simulink model "test_com_SensorFusion_SF_D4_ukf"  (R2019b)
settings: Solver=FixedStepDiscrete  StartTime=0  StopTime=stop  FixedStep=0.001  RelTol=1e-3
undefined symbols (not defined in the file or in its folder): breakpoints_camber_posZ, breakpoints_camber_RollAngle, BxTM, ByTM, camber_posZ_rear, camber_RollAngle_front, camber_RollAngle_rear, CxTM, CyTM, enable_kalman_standing, enable_simpleTireLoad_pGL, enable_v2o_direct, g, gamma_stat_front, gamma_stat_rear, gearbox_ratio, l_F, l_R, m_sprung, m_unsprung_quarter, mag_calib_front_center, mag_calib_front_compmatrix, mag_calib_rear_center, mag_calib_rear_compmatrix, should_be_in_theSensorFusion, switch_lat_accel_tireloadestimE8, switch_rocker_direction_FL, switch_rocker_direction_FR, switch_rocker_direction_RL, switch_rocker_direction_RR, switch_VelYcalculation_pSF, testStart_VelX_pSF, testVelY_pSF, tire_r_dyn, track_angle_front, track_width_front, track_width_rear, v2o_x, wheel_kinematics_breakpoints, wheel_kinematics_FL_data, wheel_kinematics_FR_data, wheelbase, x9DFrontX, x9DFrontY, x9DRearX, x9DRearY
libraries: SignalProcessingSensorFusionLib x30, simulink x9
(part 7 of 9)

== matlab function test_com_SensorFusion_SF_D4_ukf/Subsystem14/SensorFusion_E10/Sturzberechnung2/MATLAB Function ==
  data: PosZ input; Camber_PosZ_front output; Camber_PosZ_rear output
function [Camber_PosZ_front, Camber_PosZ_rear] = fcn(PosZ)
Camber_PosZ_front=max(interp1([-25 -22.50 -20.00 -17.50 -15.00 -12.50 -10.00 -7.50 ...
    -5.00 -2.50 0.00 2.50 5.00 7.50 10.00 12.50 15.00 17.50 20.00 22.50 25.00 ], ...
    [-0.83 -0.74 -0.65 -0.56 -0.47 -0.39 -0.30 -0.23 -0.15 -0.07 0.00 0.07 0.14 0.20 ...
    0.27 0.33 0.39 0.44 0.50 0.55 0.60], PosZ,'spline'));
Camber_PosZ_rear=max(interp1([-25 -22.50 -20.00 -17.50 -15.00 -12.50 -10.00 -7.50 ...
    -5.00 -2.50 0.00 2.50 5.00 7.50 10.00 12.50 15.00 17.50 20.00 22.50 25.00],...
    [-0.64 -0.57 -0.50 -0.44 -0.37 -0.30 -0.24 -0.18 -0.12 -0.06 0.00 0.06 0.11 ...
    0.17 0.22 0.27 0.32 0.37 0.41 0.46 0.50], PosZ,'spline'));

end

== matlab function test_com_SensorFusion_SF_D4_ukf/Subsystem14/SensorFusion_E10/Subsystem/TireLoadEstimationE8/tireload estimator  ==
  settings: updateMethod=DISCRETE  sampleTime=0.002
  data: u_in input single; z input single; x_hat output single; m_sprung parameter single; m_unsprung_quarter parameter single; J_Sxx parameter single; J_Syy parameter single; l_R parameter single; l_F parameter single; wheelbase parameter single; track_width_front parameter single; track_width_rear parameter single; h_aero parameter single; g parameter single; rho_air parameter single; h_cg parameter single; cdA parameter single; y output single; P_diag output single; offset output single; lp output single; clA_front parameter single; clA_rear parameter single; motion_ratio_front parameter single; motion_ratio_rear parameter single; motion_ratio_heave_front parameter single; motion_ratio_heave_rear parameter single; motion_ratio_roll_front parameter single; motion_ratio_roll_rear parameter single; spring_stiff_heave_front parameter single; spring_stiff_heave_rear parameter single; damp_coef_heave_front_push parameter single; damp_coef_heave_front_pull parameter single; damp_coef_heave_rear_push parameter single; damp_coef_heave_rear_pull parameter single; spring_stiff_roll_front parameter single; spring_stiff_roll_rear parameter single; damp_coef_roll_front_push parameter single; damp_coef_roll_front_pull parameter single; damp_coef_roll_rear_push parameter single; damp_coef_roll_rear_pull parameter single
function [x_hat, y, P_diag, offset, lp]  = fcn(u_in, z,...
                           m_sprung, m_unsprung_quarter, J_Sxx, J_Syy,...
                           l_R, l_F, wheelbase, track_width_front, track_width_rear, h_aero,...
                           g, rho_air,...
                           h_cg, cdA, clA_front, clA_rear, ...
                            motion_ratio_front, motion_ratio_rear,...
                            motion_ratio_heave_front, motion_ratio_heave_rear,...
                            motion_ratio_roll_front, motion_ratio_roll_rear,...
                           spring_stiff_heave_front, spring_stiff_heave_rear,...
                           damp_coef_heave_front_push, damp_coef_heave_front_pull,...
                           damp_coef_heave_rear_push, damp_coef_heave_rear_pull,...
                           spring_stiff_roll_front, spring_stiff_roll_rear,...
                           damp_coef_roll_front_push, damp_coef_roll_front_pull,...
                           damp_coef_roll_rear_push, damp_coef_roll_rear_pull)

% x    = [z; z_dot; phi; phi_dot; theta; theta_dot];
% u_in = [a_x; a_y; v];
% u    = [a_x; a_y; g; F_aerox; F_aeroFz; F_aeroRz];
% z    = [z; phiF; phiR; theta];
% y    = [tireloadFL; tireloadFR; tireloadRL; tireloadRR];

persistent P x t

% Initialisierung
if isempty(P)
    %Initial state / Initialwerte Zustandsvektor
    x = single([0; 0; 0; 0; 0; 0; 0; 0; 0; 0]);  
    
    %Initial uncertainty / Initialwerte Koviarianzatrix 
    P = single(diag([0; 0; 0; 0; 0; 0; 0; 0; 0; 0]));
    
    %Initial timer / Initialiserung Zähler
    t = single(0);
end

dt    = 0.001;                                 %Time step / Zeitschritt
I     = eye(10);                               %Identity matrix / Einheitsmatrix

% MonoShock Auswahl Druck/Zug-Stufe
if x(6)*l_F + x(2) < 0  %Vorne Druck
    k_msF =2759;% = damp_coef_heave_front_push;
else                    %Vorne Zug
    k_msF =3941;%= damp_coef_heave_front_pull;
end

if x(6)*l_R + x(2) > 0  %Hinten Druck
    k_msR =4137;%= damp_coef_heave_rear_pull;
else                    %Hinten Zug
    k_msR =2869;%= damp_coef_heave_rear_push;
end


% Rolldämpfer Auswahl Druck/Zug-Stufe
if x(4) < 0             % if Bedingung muss überprüft werden!
    k_rdF =1860;%= damp_coef_roll_front_push;
    k_rdR =1876;%= damp_coef_roll_rear_push;
else
    k_rdF =1860;%= damp_coef_roll_front_pull;
    k_rdR =1876;%= damp_coef_roll_rear_pull; 
end

% Aerokräfte
F_aeroFz     = 0.5 * rho_air * clA_front * u_in(3)^2 ;
F_aeroRz     = 0.5 *  rho_air * clA_rear * u_in(3)^2 ;
F_aerox      = 0.5 *  rho_air * cdA   * u_in(3)^2 ;

% Systemdynamik
a21 = -4 * ( motion_ratio_heave_front^2*spring_stiff_heave_front + motion_ratio_heave_rear^2*spring_stiff_heave_rear ) / m_sprung;
a22 = -4 * ( motion_ratio_heave_front^2*k_msF + motion_ratio_heave_front^2*k_msR ) / m_sprung;
a25 =  4 * ( l_F*motion_ratio_heave_front^2*spring_stiff_heave_front - l_R*motion_ratio_heave_rear^2*spring_stiff_heave_rear ) / m_sprung;
a26 =  4 * ( l_F*motion_ratio_heave_front^2*k_msF - l_R*motion_ratio_heave_rear^2*k_msR ) / m_sprung;
a43 = -( track_width_front^2*motion_ratio_roll_front^2*spring_stiff_roll_front + track_width_rear^2*motion_ratio_roll_rear^2*spring_stiff_roll_rear ) / J_Sxx;
a44 = -( track_width_front^2*motion_ratio_roll_front^2*k_rdF + track_width_rear^2*motion_ratio_roll_rear^2*k_rdR ) / J_Sxx;
a61 =  4 * ( l_F*motion_ratio_heave_front^2*spring_stiff_heave_front - l_R*motion_ratio_heave_rear^2*spring_stiff_heave_rear ) / J_Syy;
a62 =  4 * ( l_F*motion_ratio_heave_front^2*k_msF - l_R*motion_ratio_heave_rear^2*k_msR ) / J_Syy;
a65 = -4 * ( l_F^2*motion_ratio_heave_front^2*spring_stiff_heave_front + l_R^2*motion_ratio_heave_rear^2*spring_stiff_heave_rear ) / J_Syy;
a66 = -4 * ( l_F^2*motion_ratio_heave_front^2*k_msF + l_R^2*motion_ratio_heave_rear^2*k_msR ) / J_Syy;

A = [  0,   1,   0,   0,   0,   0,  0,   0,   0,   0;
     a21, a22,   0,   0, a25, a26,  0,   0,   0,   0;
       0,   0,   0,   1,   0,   0,  0,   0,   0,   0;
       0,   0, a43, a44,   0,   0,  0,   0,   0,   0;
       0,   0,   0,   0,   0,   1,  0,   0,   0,   0;
     a61, a62,   0,   0, a65, a66,  0,   0,   0,   0;
       0,   0,   0,   0,   0,   0,  0,   0,   0,   0;
       0,   0,   0,   0,   0,   0,  0,   0,   0,   0;
       0,   0,   0,   0,   0,   0,  0,   0,   0,   0;
       0,   0,   0,   0,   0,   0,  0,   0,   0,   0];

b25 =  1 / m_sprung;
b26 =  1 / m_sprung;
b42 =  h_cg * m_sprung / J_Sxx;
b61 = -h_cg * m_sprung / J_Syy;
b64 =  h_aero / J_Syy;
b65 = -l_F / J_Syy;
b66 =  l_R / J_Syy;

B = [  0,   0,   0,   0,   0;
       0,   0,   0, b25, b26;
       0,   0,   0,   0,   0;
       0, b42,   0,   0,   0;
       0,   0,   0,   0,   0;
     b61,   0, b64, b65, b66;
       0,   0,   0,   0,   0;
       0,   0,   0,   0,   0;
       0,   0,   0,   0,   0;
       0,   0,   0,   0,   0];                          

% RICHTUNG VON F_aerox CHECKEN!!!
u = [-u_in(1); u_in(2); -F_aerox; -F_aeroFz; -F_aeroRz];


% Measurement function / Messmatrix
H = [-1/motion_ratio_front, 0,  track_width_front/motion_ratio_front, 0,  l_F/motion_ratio_front, 0, 1, 0, 0, 0; 
     -1/motion_ratio_front, 0, -track_width_front/motion_ratio_front, 0,  l_F/motion_ratio_front, 0, 0, 1, 0, 0;
     -1/motion_ratio_rear, 0,  track_width_rear/motion_ratio_rear, 0, -l_R/motion_ratio_rear, 0, 0, 0, 1, 0;
     -1/motion_ratio_rear, 0, -track_width_rear/motion_ratio_rear, 0, -l_R/motion_ratio_rear, 0, 0, 0, 0, 1];

% Measurement noise covariance / Messrauschkovarianzmatrix
R = diag([1; 1; 1; 1]);

% Process Noise Covariance / Prozessrauschkovarianzmatrix 
if abs(u_in(3)) <= 0.5                      %keine statische Offsetzschätzung
        q_offset = 0;
elseif abs(u_in(3)) > 0.1 && t < 3          %schnelle Anfangsschätzung
        q_offset = 1e-8;
        t = t + dt;
else                                        %langsame Detailanpassung
        q_offset = 1e-16;
end
Q = diag([1e-9; 1e-9; 1e-9; 1e-9; 6e-9; 6e-9; q_offset; q_offset; q_offset; q_offset]);

% Prädiktorschritt
x = x + dt * ( A * x + B * u );
P = ( I + dt * A ) * P * ( I + dt * A )' + Q;

% Korrektorschritt
K = P * H' / ( H * P * H' + R );            %Filter-Matrix (Kalman-Gain)
x = x + K * ( z - H * x );                  %aktualisieren des Systemzustands
P = ( I - K * H ) * P;                      %aktualisieren der Kovarianz

% Ausgang
C = [2*motion_ratio_heave_front^2*spring_stiff_heave_front, 2*motion_ratio_heave_front^2*k_msF, -track_width_front*motion_ratio_roll_front^2*spring_stiff_roll_front, -track_width_front*motion_ratio_roll_front^2*k_rdF, -2*l_F*motion_ratio_heave_front^2*spring_stiff_heave_front, -2*l_F*motion_ratio_heave_front^2*k_msF, 0, 0, 0, 0;
     2*motion_ratio_heave_front^2*spring_stiff_heave_front, 2*motion_ratio_heave_front^2*k_msF,  track_width_front*motion_ratio_roll_front^2*spring_stiff_roll_front,  track_width_front*motion_ratio_roll_front^2*k_rdF, -2*l_F*motion_ratio_heave_front^2*spring_stiff_heave_front, -2*l_F*motion_ratio_heave_front^2*k_msF, 0, 0, 0, 0;
     2*motion_ratio_heave_rear^2*spring_stiff_heave_rear, 2*motion_ratio_heave_rear^2*k_msR, -track_width_rear*motion_ratio_roll_rear^2*spring_stiff_roll_rear, -track_width_rear*motion_ratio_roll_rear^2*k_rdR,  2*l_R*motion_ratio_heave_rear^2*spring_stiff_heave_rear,  2*l_R*motion_ratio_heave_rear^2*k_msR, 0, 0, 0, 0;
     2*motion_ratio_heave_rear^2*spring_stiff_heave_rear, 2*motion_ratio_heave_rear^2*k_msR,  track_width_rear*motion_ratio_roll_rear^2*spring_stiff_roll_rear,  track_width_rear*motion_ratio_roll_rear^2*k_rdR,  2*l_R*motion_ratio_heave_rear^2*spring_stiff_heave_rear,  2*l_R*motion_ratio_heave_rear^2*k_msR, 0, 0, 0, 0];

D = [m_unsprung_quarter + 0.5*m_sprung*l_R/wheelbase; 
     m_unsprung_quarter + 0.5*m_sprung*l_R/wheelbase; 
     m_unsprung_quarter + 0.5*m_sprung*l_F/wheelbase; 
     m_unsprung_quarter + 0.5*m_sprung*l_F/wheelbase]*g;

y = C * x + D;

% Begrenzung der Radlast
for n=1:1:4
    if y(n) > 1800
        y(n) = 1800;
    elseif y(n) < 0
        y(n) = 0;
    end
end

% Ausgabe
os_z     = - 0.5*(motion_ratio_front*x(7)+motion_ratio_front*x(8))*l_R/wheelbase - 0.5*(motion_ratio_rear*x(9)+motion_ratio_rear*x(10))*l_F/wheelbase;  
os_phi  = l_R/wheelbase*( x(7)*motion_ratio_front - x(8)*motion_ratio_front ) / track_width_front + l_F/wheelbase*( x(9)*motion_ratio_rear - x(10)*motion_ratio_rear ) / track_width_rear;
os_theta = ( motion_ratio_front*x(7) + motion_ratio_front*x(8) - motion_ratio_rear*x(9) - motion_ratio_rear*x(10) ) / 2 * wheelbase;

x_hat  = [ x(1) + os_z;
           x(2);
          (x(3) + os_phi)   * 180 / pi;
           x(4)             * 180 / pi;
          (x(5) + os_theta) * 180 / pi;
           x(6)             * 180 / pi];

P_diag = [P(1,1), P(2,2), P(3,3), P(4,4), P(5,5), P(6,6), P(7,7), P(8,8), P(9,9), P(10,10)];
offset = [x(7); x(8); x(9); x(10)];
lp = H * x;

end

== matlab function test_com_SensorFusion_SF_D4_ukf/Subsystem14/SensorFusion_E10/Sturzberechnung2/MATLAB Function1 ==
  data: Camber_RollAngle_front output; Camber_RollAngle_rear output; RollAngle input
function [Camber_RollAngle_front, Camber_RollAngle_rear]= fcn (RollAngle)
Camber_RollAngle_front=max(interp1([-1.50 -1.35 -1.20 -1.05 -0.90 -0.75 -0.60 -0.45 -0.30 -0.15 0.00 ...
0.15 0.30 0.45 0.60 0.75 0.90 1.05 1.20 1.35 1.50], ...
    [1.02 0.92 0.82 0.72 0.62 0.52 0.42 0.31 0.21 0.11 0.00 -0.11 -0.21 -0.32 -0.43 -0.53 -0.64 ...
-0.75 -0.86 -0.97 -1.08], RollAngle,'spline'));
Camber_RollAngle_rear=max(interp1([-1.50 -1.35 -1.20 -1.05 -0.90 -0.75 -0.60 -0.45 -0.30 -0.15 0.00 ...
0.15 0.30 0.45 0.60 0.75 0.90 1.05 1.20 1.35 1.50],...
    [1.11 1.00 0.89 0.78 0.67 0.56 0.45 0.34 0.23 0.11 0.00 -0.12 -0.23 -0.35 -0.46 -0.58 ...
-0.70 -0.81 -0.93 -1.05 -1.17], RollAngle,'spline'));
end

== matlab function test_com_SensorFusion_SF_D4_ukf/Subsystem14/SensorFusion_E10/Subsystem/simpleTireLoadEstimation/MATLAB Function ==
  data: a_x input; F_z_vl output; a_y input; F_z_vr output; F_z_hl output; F_z_hr output
function [F_z_vl, F_z_vr, F_z_hl, F_z_hr] = Radlast_Beschleunigung_e9_SAE(a_x, a_y)
m=240;
g=9.81;
l=1.540;
l_v=0.796;
l_h=l-l_v;
h_s=0.2648;
b_v=0.6*2;
b_h=0.6*2;
F_z_vl=single(0);
F_z_vr=single(0);
F_z_hl=single(0);
F_z_hr=single(0);
 %m=Fahrzeugmasse; h_s= Schwerpunktshöhe (von SP zu Anbindung von Rods an Radträger); l_h= Abstand von HA zu
 %SP; l_v=Radstand von VA zum SP l=Radstand; a_x=Beschleunigung in x-Richtung; a_y=Beschleunigung
 %in y-Richtung; b_v=Spurbreite vorne;b_h=Spurbreite hinten; 
 
 %EDITIERT, so dass Vorzeichen vor h_s*a_y/(b_v*g) jeweils getauscht wurde

m_ges_f= m * (l-l_v)/l;
m_ges_r= m * l_v/l;
Delta_TireLoad_x = m * (h_s/(2*l))*a_x; %die 2 hier ist in E7 Radlastschätzer nicht so drin
%{ TireLoad = [...
%    m_ges_f *(0.5*g + (h_s/b_v)* a_y) - Delta_TireLoad_x ...
%    m_ges_f *(0.5*g - (h_s/b_v)* a_y) - Delta_TireLoad_x ...
%    m_ges_r *(0.5*g + (h_s/b_h)* a_y) + Delta_TireLoad_x ...
%    m_ges_r *(0.5*g - (h_s/b_h)* a_y) + Delta_TireLoad_x];
%}

SiL_WheelStates = [ ...
    m*(l_h*g-h_s*a_x)*(0.5+(h_s*a_y/(b_v*g)))/l;
    m*(l_h*g-h_s*a_x)*(0.5-(h_s*a_y/(b_v*g)))/l;
    m*(l_v*g+h_s*a_x)*(0.5+(h_s*a_y/(b_h*g)))/l;
    m*(l_v*g+h_s*a_x)*(0.5-(h_s*a_y/(b_h*g)))/l
    ];
if SiL_WheelStates(1)<0
    F_z_vl = single(0);
else
    F_z_vl = SiL_WheelStates(1);
end

if SiL_WheelStates(2)<0
    F_z_vr = single(0);
else
    F_z_vr = SiL_WheelStates(2);
end

if SiL_WheelStates(3)<0
    F_z_hl = single(0);
else
    F_z_hl = SiL_WheelStates(3);
end

if SiL_WheelStates(4)<0
    F_z_hr = single(0);
else
    F_z_hr = SiL_WheelStates(4);
end

end

== matlab function test_com_SensorFusion_SF_D4_ukf/Subsystem14/SensorFusion_E10/TireModel_simplePacejka1 ==
  data: TireLoad input; TireSlipLong input; TireLoadEff output; TireForceLong output; TireSlipAngle input; mux_nominal input; TireForceLat output; l_F parameter; l_R parameter; wheelbase parameter; m_unsprung_quarter parameter; m_sprung parameter; BxTM parameter; ByTM parameter; CyTM parameter; CxTM parameter; g parameter
function [TireLoadEff, TireForceLong, TireForceLat] = TireModel_simplePacejka(TireLoad, TireSlipLong, TireSlipAngle, ...
    mux_nominal, l_F, l_R, wheelbase, m_unsprung_quarter, m_sprung, BxTM, ByTM, CyTM, CxTM, g)
%% set variables
Fz = TireLoad;
s_long = TireSlipLong;
s_lat = tan(TireSlipAngle); % sin???
dim_wheel = size(TireLoad);

Fx_eff = zeros(dim_wheel);
Fy_eff = zeros(dim_wheel);
Fxy_res  = zeros(dim_wheel);

e = 0.001;

%% set parameters

ez = 0.05; %0.05 richtwert dictonary
mu_x = mux_nominal;   % aus settings herführen
mu_y = 1.6;   % oder eins? 


%% calculate 
s_res = sqrt(s_long.^2 + s_lat.^2); % nominated total tire slips

Fznull_FL= 0.5*g*l_R/wheelbase*m_sprung+g*m_unsprung_quarter;
Fznull_FR= 0.5*g*l_R/wheelbase*m_sprung+g*m_unsprung_quarter;
Fznull_RL= 0.5*g*l_F/wheelbase*m_sprung+g*m_unsprung_quarter;
Fznull_RR= 0.5*g*l_F/wheelbase*m_sprung+g*m_unsprung_quarter;
Fz0=[Fznull_FL; Fznull_FR; Fznull_RL; Fznull_RR];

Fz_eff = Fz.*(1-ez*(Fz./Fz0).^2); % effective tire loads for mu
Dx = Fz_eff*mu_x; % D-terms for long. in Pacejka
Dy = Fz_eff*mu_y; % D-terms for lat. in Pacejka

Fx_stat = Fz_eff*mu_x.* sin( CxTM* atan(BxTM*s_res./mu_x) ); % pure long. tire forces
Fy_stat = Fz_eff*mu_y.* sin( CyTM* atan(ByTM*s_res./mu_y) ); % pure lat. tire forces
% Fx_stat = D_*sin( C_ * atan(B_*s_ - E_*(B_*s_-atan(B_*s_))) ) - sv;
% Fx_stat = D_*sin( C_ * atan(B_*s_ - E_*(B_*s_-atan(B_*s_))) ) - sv;

% combine long. lat. forces
for i = 1:numel(TireLoad)
    if s_res(i) == 0
        Fx_eff(i) = 0;
        Fy_eff(i) = 0;
    else
        Fxy_res(i) = sqrt( (s_long(i)^2*Fx_stat(i)^2+s_lat(i)^2*Fy_stat(i)^2)/(s_res(i)^2) );
        Fx_eff(i) = Fxy_res(i) *(s_long(i)/s_res(i)); % effective long. tire forces
        Fy_eff(i) = Fxy_res(i) *(s_lat(i)/s_res(i)); % effective lat. tire forces
    end
end

% Fxy_res = Fz_eff*mu;

TireLoadEff = single(Fz_eff);
TireForceLong = single(Fx_eff);
TireForceLat = single(Fy_eff);
end

== matlab function test_com_SensorFusion_SF_D4_ukf/Subsystem14/SensorFusion_E10/simpleTireLoadEstimation/MATLAB Function ==
  data: a_x input; F_z_vl output; a_y input; F_z_vr output; F_z_hl output; F_z_hr output
function [F_z_vl, F_z_vr, F_z_hl, F_z_hr] = Radlast_Beschleunigung_e9_SAE(a_x, a_y)
m=240;
g=9.81;
l=1.540;
l_v=0.796;
l_h=l-l_v;
h_s=0.2648;
b_v=0.6*2;
b_h=0.6*2;
F_z_vl=single(0);
F_z_vr=single(0);
F_z_hl=single(0);
F_z_hr=single(0);
 %m=Fahrzeugmasse; h_s= Schwerpunktshöhe (von SP zu Anbindung von Rods an Radträger); l_h= Abstand von HA zu
 %SP; l_v=Radstand von VA zum SP l=Radstand; a_x=Beschleunigung in x-Richtung; a_y=Beschleunigung
 %in y-Richtung; b_v=Spurbreite vorne;b_h=Spurbreite hinten; 
 
 %EDITIERT, so dass Vorzeichen vor h_s*a_y/(b_v*g) jeweils getauscht wurde

m_ges_f= m * (l-l_v)/l;
m_ges_r= m * l_v/l;
Delta_TireLoad_x = m * (h_s/(2*l))*a_x; %die 2 hier ist in E7 Radlastschätzer nicht so drin
%{ TireLoad = [...
%    m_ges_f *(0.5*g + (h_s/b_v)* a_y) - Delta_TireLoad_x ...
%    m_ges_f *(0.5*g - (h_s/b_v)* a_y) - Delta_TireLoad_x ...
%    m_ges_r *(0.5*g + (h_s/b_h)* a_y) + Delta_TireLoad_x ...
%    m_ges_r *(0.5*g - (h_s/b_h)* a_y) + Delta_TireLoad_x];
%}

SiL_WheelStates = [ ...
    m*(l_h*g-h_s*a_x)*(0.5+(h_s*a_y/(b_v*g)))/l;
    m*(l_h*g-h_s*a_x)*(0.5-(h_s*a_y/(b_v*g)))/l;
    m*(l_v*g+h_s*a_x)*(0.5+(h_s*a_y/(b_h*g)))/l;
    m*(l_v*g+h_s*a_x)*(0.5-(h_s*a_y/(b_h*g)))/l
    ];
if SiL_WheelStates(1)<0
    F_z_vl = single(0);
else
    F_z_vl = SiL_WheelStates(1);
end

if SiL_WheelStates(2)<0
    F_z_vr = single(0);
else
    F_z_vr = SiL_WheelStates(2);
end

if SiL_WheelStates(3)<0
    F_z_hl = single(0);
else
    F_z_hl = SiL_WheelStates(3);
end

if SiL_WheelStates(4)<0
    F_z_hr = single(0);
else
    F_z_hr = SiL_WheelStates(4);
end

end

== matlab function test_com_SensorFusion_SF_D4_ukf/Subsystem14/SensorFusion_E10/SensorFusion_E10/Subsystem2/9D_front_measure/MATLAB Function ==
  data: AccX_Sq input; VD_diag_9Dfront output; AccY_Sq input; AccZ_Sq input; RollRate_Sq input; PitchRate_Sq input; YawRate_Sq input

function VD_diag_9Dfront = diag(AccX_Sq, AccY_Sq, AccZ_Sq, RollRate_Sq, PitchRate_Sq, YawRate_Sq)
bad_Sq_counter=single(0);
VD_diag_9Dfront=0;
persistent timestep_counter_old
if isempty(timestep_counter_old)
    timestep_counter_old=0;
end


if AccX_Sq>4
    bad_Sq_counter=bad_Sq_counter+1;
end
if AccY_Sq>4
    bad_Sq_counter=bad_Sq_counter+1;
end
if AccZ_Sq>4
    bad_Sq_counter=bad_Sq_counter+1;
end
if YawRate_Sq>4
    bad_Sq_counter=bad_Sq_counter+1;
end
if RollRate_Sq>4
    bad_Sq_counter=bad_Sq_counter+1;
end
if PitchRate_Sq>4
    bad_Sq_counter=bad_Sq_counter+1;
end

if  bad_Sq_counter>3
    timestep_counter=timestep_counter_old+1;
else 
    timestep_counter=0;
end
if bad_Sq_counter>3 && timestep_counter >4
    VD_diag_9Dfront=1;
end

timestep_counter_old=timestep_counter;

end

== matlab function test_com_SensorFusion_SF_D4_ukf/Subsystem14/SensorFusion_E10/SensorFusion_E10/Subsystem2/9D_rear_measure/MATLAB Function ==
  data: AccX_Sq input; VD_diag_9Drear output; AccY_Sq input; AccZ_Sq input; YawRate_Sq input; PitchRate_Sq input; RollRate_Sq input
function VD_diag_9Drear = diag(AccX_Sq, AccY_Sq, AccZ_Sq, YawRate_Sq, PitchRate_Sq, RollRate_Sq)
bad_Sq_counter=single(0);
VD_diag_9Drear=0;
persistent timestep_counter_old
if isempty(timestep_counter_old)
    timestep_counter_old=0;
end


if AccX_Sq>4
    bad_Sq_counter=bad_Sq_counter+1;
end
if AccY_Sq>4
    bad_Sq_counter=bad_Sq_counter+1;
end
if AccZ_Sq>4
    bad_Sq_counter=bad_Sq_counter+1;
end
if YawRate_Sq>4
    bad_Sq_counter=bad_Sq_counter+1;
end
if RollRate_Sq>4
    bad_Sq_counter=bad_Sq_counter+1;
end
if PitchRate_Sq>4
    bad_Sq_counter=bad_Sq_counter+1;
end

if  bad_Sq_counter>3
    timestep_counter=timestep_counter_old+1;
else 
    timestep_counter=0;
end


if bad_Sq_counter>3 && timestep_counter >4
    VD_diag_9Drear=1;
end

timestep_counter_old=timestep_counter;

end

== matlab function test_com_SensorFusion_SF_D4_ukf/Subsystem14/SensorFusion_E10/SensorFusion_E10/Subsystem2/MATLAB Function1 ==
  data: VD_diag_9Dfront input; sensorFail output boolean; VD_diag_9Drear input; VD_diag_v2o input; VD_diag_RockerAngle input
function sensorFail = fcn(VD_diag_9Dfront, VD_diag_9Drear, VD_diag_v2o, VD_diag_RockerAngle)
sensorFail=false;
if VD_diag_9Dfront==1 || VD_diag_9Drear==1 || VD_diag_v2o==1 || VD_diag_RockerAngle==1
    sensorFail=true;
end 
end

== matlab function test_com_SensorFusion_SF_D4_ukf/Subsystem14/SensorFusion_E10/SensorFusion_E10/Subsystem2/RockerAngle_measure/MATLAB Function ==
  data: RockerAngle_FL_Sq input; VD_diag_RockerAngle output; RockerAngle_FR_Sq input; RockerAngle_RL_Sq input; RockerAngle_RR_Sq input
function VD_diag_RockerAngle  = diag(RockerAngle_FL_Sq, RockerAngle_FR_Sq, RockerAngle_RL_Sq, RockerAngle_RR_Sq)
bad_Sq_counter=single(0);
VD_diag_RockerAngle=0;
persistent timestep_counter_old
if isempty(timestep_counter_old)
    timestep_counter_old=0;
end

if RockerAngle_FL_Sq>4
    bad_Sq_counter=bad_Sq_counter+1;
end
if RockerAngle_FR_Sq>4
    bad_Sq_counter=bad_Sq_counter+1;
end
if RockerAngle_RL_Sq>4
    bad_Sq_counter=bad_Sq_counter+1;
end
if RockerAngle_RR_Sq>4
    bad_Sq_counter=bad_Sq_counter+1;
end

if  bad_Sq_counter>1
    timestep_counter=timestep_counter_old+1;
else 
    timestep_counter=0;
end

if bad_Sq_counter>0 && timestep_counter >8
    VD_diag_RockerAngle=1;
end

timestep_counter_old=timestep_counter;
end
